simulink model "inverter"  (R2020a)
settings: Solver=VariableStepAuto  StartTime=0.0  StopTime=0.1  RelTol=1e-3
model workspace (MAT data in the model file):
  f_tri = Simulink.Parameter
  f_tri.Value = 1650
  f_tri.DataType = 'auto'
  f_tri.Dimensions = [1 1]
  m_a = 0.8
  m_f = Simulink.Parameter
  m_f.Value = 33
  m_f.DataType = 'auto'
  m_f.Dimensions = [1 1]
libraries: powerlib x11, simulink x3, powerlib_meascontrol x1
settings Model: OrderedModelArguments=off  Creator=albertinagalan  LastModifiedBy=albertinagalan

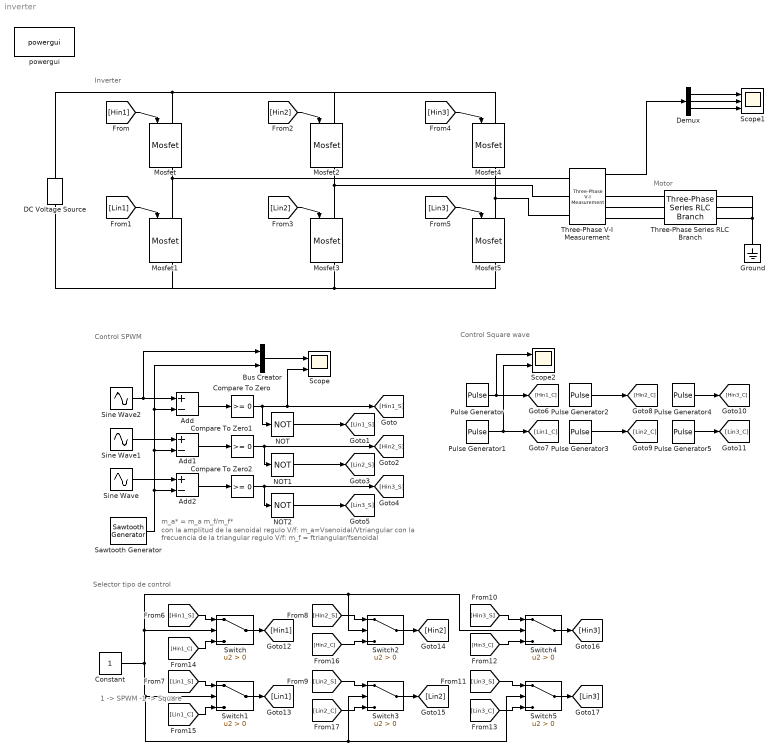
== system inverter ==
  note: m_a* = m_a m_f/m_f*
  note: Selector tipo de control
  note: 1  -> SPWM
      | -1 -> Square
  note: Control Square wave
  note: Control SPWM
  note: Motor
  note: Inverter
  note: con la amplitud de la senoidal regulo V/f: m_a=Vsenoidal/Vtriangular
      | con la frecuencia de la triangular regulo V/f: m_f = ftriangular/fsenoidal
  Add : Sum  Inputs=+-
  Add1 : Sum  Inputs=+-
  Add2 : Sum  Inputs=+-
  Bus Creator : BusCreator  Inputs=2
  Compare To Zero : simulink/Logic and Bit Operations/Compare To Zero  relop=>=  OutDataTypeStr=boolean
  Compare To Zero1 : simulink/Logic and Bit Operations/Compare To Zero  relop=>=  OutDataTypeStr=boolean
  Compare To Zero2 : simulink/Logic and Bit Operations/Compare To Zero  relop=>=  OutDataTypeStr=boolean
  Constant : Constant
  DC Voltage Source : powerlib/Electrical Sources/DC Voltage Source  Amplitude=100  Measurements=None
  Demux : Demux  Outputs=3
  Ground : powerlib/Elements/Ground  LConnTagsString=a
  Mosfet{,1..5} (6 alike) : powerlib/Power Electronics/Mosfet  Ron=0.1  Lon=0  Rd=0.01  Vfd=0  IC=0  Rs=1e5  Cs=inf  Measurements=on
  NOT : Logic  Operator=NOT  IconShape=distinctive  AllPortsSameDT=off  OutDataTypeStr=boolean
  NOT1 : Logic  Operator=NOT  IconShape=distinctive  AllPortsSameDT=off  OutDataTypeStr=boolean
  NOT2 : Logic  Operator=NOT  IconShape=distinctive  AllPortsSameDT=off  OutDataTypeStr=boolean
  Pulse Generator : DiscretePulseGenerator  PulseType=Time based  Period=0.02  PulseWidth=50
  Pulse Generator1 : DiscretePulseGenerator  PulseType=Time based  Period=0.02  PulseWidth=50  PhaseDelay=(180*0.02)/360
  Pulse Generator2 : DiscretePulseGenerator  PulseType=Time based  Period=0.02  PulseWidth=50  PhaseDelay=(120*0.02)/360
  Pulse Generator3 : DiscretePulseGenerator  PulseType=Time based  Period=0.02  PulseWidth=50  PhaseDelay=(300*0.02)/360
  Pulse Generator4 : DiscretePulseGenerator  PulseType=Time based  Period=0.02  PulseWidth=50  PhaseDelay=(240*0.02)/360
  Pulse Generator5 : DiscretePulseGenerator  PulseType=Time based  Period=0.02  PulseWidth=50  PhaseDelay=(60*0.02)/360
  Sawtooth Generator : powerlib_meascontrol/Pulse & Signal Generators/Sawtooth Generator  Freq=f_tri  Phase=180  Ts=0
  Scope : Scope  NumInputPorts=2
  Scope1 : Scope  NumInputPorts=3
  Scope2 : Scope  NumInputPorts=2
  Sine Wave : Sin  Amplitude=m_a  Frequency=f_tri/m_f*2*pi  Phase=4/3*pi  SampleTime=0
  Sine Wave1 : Sin  Amplitude=m_a  Frequency=f_tri/m_f*2*pi  Phase=2/3*pi  SampleTime=0
  Sine Wave2 : Sin  Amplitude=m_a  Frequency=f_tri/m_f*2*pi  SampleTime=0
  Switch{,1..5} (6 alike) : Switch  Criteria=u2 > Threshold
  Three-Phase Series RLC Branch : powerlib/Elements/Three-Phase Series RLC Branch  LConnTagsString=A|B|C  RConnTagsString=A|B|C  BranchType=RL  Resistance=20  Inductance=1e-3  Capacitance=1e-6  Measurements=None
  Three-Phase V-I Measurement : powerlib/Measurements/Three-Phase V-I Measurement  VoltageMeasurement=phase-to-ground  SetLabelV=off  LabelV=Vabc  Vpu=off  VpuLL=off  CurrentMeasurement=yes  SetLabelI=off  LabelI=Iabc  Ipu=off  Pbase=100e6  Vbase=500e3  OutputType=Complex  PhasorSimulation=off  PSBequivalent=0
  powergui : powerlib/powergui  Priority=1  SimulationMode=Continuous  SampleTime=50e-6  frequency=60  Iterations=50  frequencyindice=0  Pbase=100e6  ErrMax=1e-4  UnitsV=kV  UnitsW=MW  buscounter=0  FunctionMessages=off  echomessages=off  EnableUseOfTLC=off  CurrentSourceSwitches=off  DisableSnubberDevices=off  DisableRonSwitches=off  DisableVfSwitches=off  DisplayEquations=off  AutomaticDiscreteSolvers=off  SolverType=Tustin/Backward Euler (TBE)  Interpol=off  ExternalGateDelay=off  methode=off  Ts=100  x0status=blocks  SPID=on  SwTol=0  HookPort=off  NonlinearTolerance=1e-4  nMaxIteration=100  ContinueOnMaxIteration=off  RestoreLinks=warning  ResistiveCurrentMeasurement=off  Frange=[0:2:500]  Ylog=off  Xlog=on  ShowGrid=off  save=off  variable=ZData  structure=0  ZoomFFT=off  StartTime=0.0  cycles=1  DisplayStyle=1  fundamental=60  FreqAxis=off  MaxFrequency=1000  frequencyindicesteady=1  RmsSteady=1  display=off
  wires:
  Sine Wave2/1 -> Add/1, Bus Creator/1
  Sine Wave1/1 -> Add1/1
  Sine Wave/1 -> Add2/1
  Sawtooth Generator/1 -> Add2/2, Add1/2, Add/2, Bus Creator/2
  Add/1 -> Compare To Zero/1
  Add1/1 -> Compare To Zero1/1
  Add2/1 -> Compare To Zero2/1
  Bus Creator/1 -> Scope/1
  Compare To Zero/1 -> NOT/1, [Hin1_S], Scope/2
  Compare To Zero2/1 -> NOT2/1, [Hin3_S]
  Compare To Zero1/1 -> NOT1/1, [Hin2_S]
  NOT/1 -> [Lin1_S]
  NOT1/1 -> [Lin2_S]
  NOT2/1 -> [Lin3_S]
  [Lin3] -> Mosfet5/1
  [Hin3] -> Mosfet4/1
  [Lin2] -> Mosfet3/1
  [Hin2] -> Mosfet2/1
  [Hin1] -> Mosfet/1
  [Lin1] -> Mosfet1/1
  Three-Phase V-I Measurement/1 -> Demux/1
  Demux/1 -> Scope1/1
  Demux/2 -> Scope1/2
  Demux/3 -> Scope1/3
  Pulse Generator/1 -> [Hin1_C], Scope2/1
  Pulse Generator1/1 -> [Lin1_C], Scope2/2
  Pulse Generator2/1 -> [Hin2_C]
  Pulse Generator3/1 -> [Lin2_C]
  Pulse Generator4/1 -> [Hin3_C]
  Pulse Generator5/1 -> [Lin3_C]
  Switch/1 -> [Hin1]
  Switch2/1 -> [Hin2]
  [Hin3_S] -> Switch4/1
  Switch4/1 -> [Hin3]
  Switch5/1 -> [Lin3]
  [Hin1_S] -> Switch/1
  [Hin1_C] -> Switch/3
  [Lin1_S] -> Switch1/1
  [Lin1_C] -> Switch1/3
  [Hin2_S] -> Switch2/1
  [Hin2_C] -> Switch2/3
  [Lin2_S] -> Switch3/1
  [Lin2_C] -> Switch3/3
  [Hin3_C] -> Switch4/3
  [Lin3_S] -> Switch5/1
  [Lin3_C] -> Switch5/3
  Constant/1 -> Switch2/2, Switch4/2, Switch/2, Switch3/2, Switch5/2, Switch1/2
  Switch1/1 -> [Lin1]
  Switch3/1 -> [Lin2]
  connections:
  Mosfet/RConn1 -- Mosfet1/LConn1 -- Three-Phase V-I Measurement/LConn1
  Mosfet2/RConn1 -- Three-Phase V-I Measurement/LConn2 -- Mosfet3/LConn1
  Mosfet4/RConn1 -- Three-Phase V-I Measurement/LConn3 -- Mosfet5/LConn1
  DC Voltage Source/RConn1 -- Mosfet2/LConn1 -- Mosfet4/LConn1 -- Mosfet/LConn1
  Mosfet5/RConn1 -- Mosfet3/RConn1 -- Mosfet1/RConn1 -- DC Voltage Source/LConn1
  Three-Phase Series RLC Branch/LConn1 -- Three-Phase V-I Measurement/RConn1
  Three-Phase Series RLC Branch/LConn2 -- Three-Phase V-I Measurement/RConn2
  Three-Phase Series RLC Branch/LConn3 -- Three-Phase V-I Measurement/RConn3
  Three-Phase Series RLC Branch/RConn2 -- Three-Phase Series RLC Branch/RConn1 -- Three-Phase Series RLC Branch/RConn3 -- Ground/LConn1
